simulink model "single_phase_five_level_CHB"  (R2022b)
settings: Solver=ode45  StartTime=0.0  StopTime=0.02  MaxStep=1e-5  RelTol=1e-4  EnableMultiTasking=on
libraries: spsIGBTDiodeLib x8, simulink x4, spsDCVoltageSourceLib x2, spsCurrentMeasurementLib x1, spsSeriesRLCBranchLib x1, spsTHDLib x1, spsVoltageMeasurementLib x1, sps_lib x1
settings Model: Creator=OLIVIA  LastModifiedBy=ugochukwu
settings SolverCC: AlgebraicLoopSolver=TrustRegion
settings DataIOCC: LimitDataPoints=on  SaveFormat=Array  ReturnWorkspaceOutputs=off
settings OptimizationCC: LifeSpan=inf
settings DebuggingCC: SolverPrmCheckMsg=warning  UnconnectedInputMsg=warning  UnconnectedOutputMsg=warning  UnconnectedLineMsg=warning  SFUnexpectedBacktrackingDiag=warning  SFNoUnconditionalDefaultTransitionDiag=warning  SFExecutionAtInitializationDiag=none  SFMachineParentedDataDiag=warning  ArithmeticOperatorsInVariantConditions=warning
settings HardwareCC: ProdBitPerPointer=32  ProdBitPerSizeT=32  ProdBitPerPtrDiffT=32  ProdLargestAtomicFloat=None  ProdIntDivRoundTo=Undefined  ProdEndianess=Unspecified  ProdWordSize=32  ProdHWDeviceType=32-bit Generic
settings ModelReferenceCC: PropagateSignalLabelsOutOfModel=off
settings SFSimCC: SimUseLocalCustomCode=off  CustomCodeUndefinedFunction=UseInterfaceOnly
settings RTWCC: RTWUseLocalCustomCode=off
settings CodeAppCC: StateflowObjectComments=on
settings GRTTargetCC: TargetLangStandard=C89/C90 (ANSI)
settings ConfigComp: CovMetricSettings=dw  CovSaveCumulativeToWorkspaceVar=on  CovSaveSingleToWorkspaceVar=on  CovExternalEMLEnable=off  CovSFcnEnable=off
settings SimscapeCC: SimscapeNormalizeSystem=off

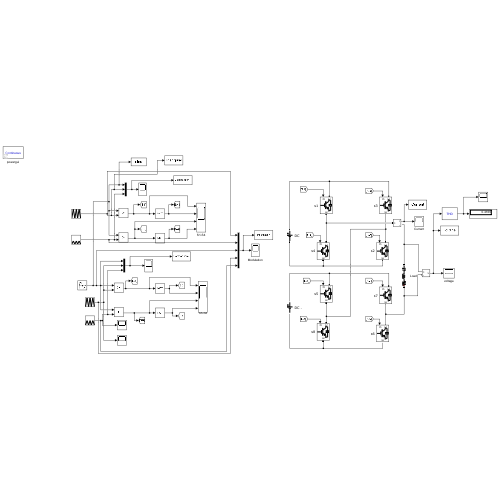
[thumbnail: Simulink's stored preview of the top-level diagram]
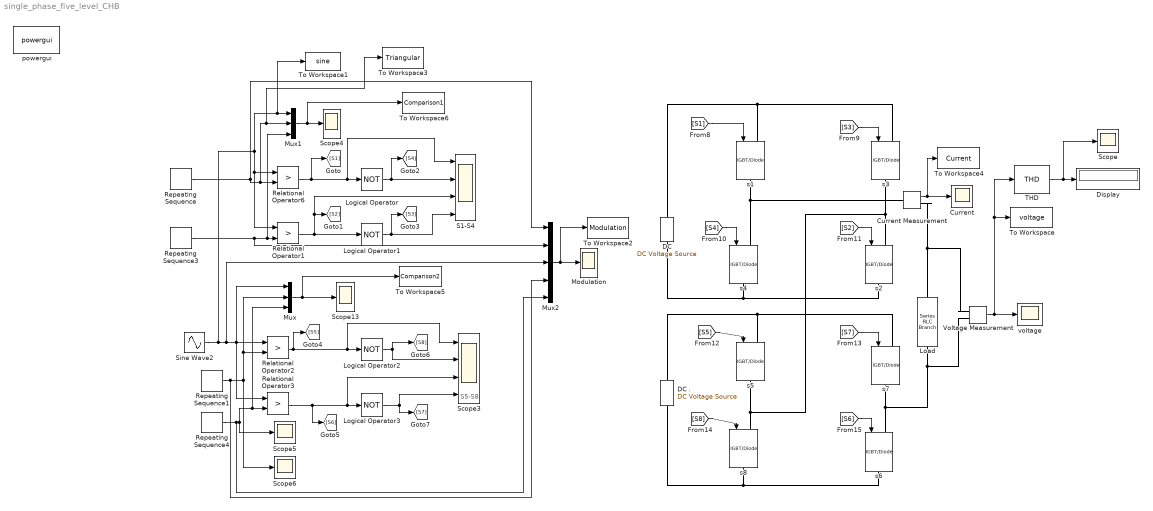
== system single_phase_five_level_CHB ==
  note: S5-S8
  Current : Scope
  Current Measurement : spsCurrentMeasurementLib/Current Measurement  PhasorSimulation=off  OutputType=Complex  PSBequivalent=0
  DC : spsDCVoltageSourceLib/DC Voltage Source  Amplitude=110  Measurements=None
  DC . : spsDCVoltageSourceLib/DC Voltage Source  Amplitude=110  Measurements=None
  Display : Display
  Load : spsSeriesRLCBranchLib/Series RLC Branch  LConnTagsString=__new0  RConnTagsString=__new0  BranchType=RLC  Resistance=100  Inductance=2e-3  SetiL0=off  InitialCurrent=0  Capacitance=1e-6  Setx0=off  InitialVoltage=0  Measurements=Branch voltage
  Logical Operator{,1..3} (4 alike) : Logic  Operator=NOT  AllPortsSameDT=off  OutDataTypeStr=boolean
  Modulation : Scope
  Mux : Mux  Inputs=3
  Mux1 : Mux  Inputs=3
  Mux2 : Mux  Inputs=5
  Relational Operator{1..3,6} (4 alike) : RelationalOperator  Operator=>  OutDataTypeStr=boolean  InputSameDT=off
  Repeating Sequence : simulink/Sources/Repeating Sequence  rep_seq_t=[0 1/4000 1/2000]  rep_seq_y=[1 1.5 1 ]
  Repeating Sequence1 : simulink/Sources/Repeating Sequence  rep_seq_t=[0 1/4000 1/2000]  rep_seq_y=[0.5 1 0.5]
  Repeating Sequence3 : simulink/Sources/Repeating Sequence  rep_seq_t=[0 1/4000 1/2000]  rep_seq_y=[-1.5 -1 -1.5 ]
  Repeating Sequence4 : simulink/Sources/Repeating Sequence  rep_seq_t=[0 1/4000 1/2000]  rep_seq_y=[-1 -0.5 -1]
  S1-S4 : Scope  NumInputPorts=4
  Scope{,4..6,13} (5 alike) : Scope
  Scope3 : Scope  NumInputPorts=4
  Sine Wave2 : Sin  Amplitude=1.4  Frequency=2*50*pi  SampleTime=0
  THD : spsTHDLib/THD  Freq=50  Ts=0
  To Workspace : ToWorkspace  VariableName=voltage  SaveFormat=Timeseries  SampleTime=-1
  To Workspace1 : ToWorkspace  VariableName=sine  SaveFormat=Timeseries  SampleTime=-1
  To Workspace2 : ToWorkspace  VariableName=Modulation  SaveFormat=Timeseries  SampleTime=-1
  To Workspace3 : ToWorkspace  VariableName=Triangular  SaveFormat=Timeseries  SampleTime=-1
  To Workspace4 : ToWorkspace  VariableName=Current  SaveFormat=Timeseries  SampleTime=-1
  To Workspace5 : ToWorkspace  VariableName=Comparison2  SaveFormat=Timeseries  SampleTime=-1
  To Workspace6 : ToWorkspace  VariableName=Comparison1  SaveFormat=Timeseries  SampleTime=-1
  Voltage Measurement : spsVoltageMeasurementLib/Voltage Measurement  PhasorSimulation=off  OutputType=Complex  PSBequivalent=0
  powergui : sps_lib/powergui  Priority=1  SimulationMode=Continuous  SampleTime=50e-6  frequency=60  Iterations=50  frequencyindice=0  Pbase=100e6  ErrMax=1e-4  UnitsV=kV  UnitsW=MW  buscounter=0  FunctionMessages=off  echomessages=off  EnableUseOfTLC=off  CurrentSourceSwitches=on  DisableSnubberDevices=off  DisableRonSwitches=off  DisableVfSwitches=off  DisplayEquations=off  AutomaticDiscreteSolvers=off  SolverType=Tustin  Interpol=off  ExternalGateDelay=off  methode=off  Ts=0  x0status=blocks  SPID=off  SwTol=0  HookPort=off  NonlinearTolerance=1e-4  nMaxIteration=100  ContinueOnMaxIteration=off  RestoreLinks=warning  ResistiveCurrentMeasurement=off  Frange=[0:2:500]  Ylog=off  Xlog=on  ShowGrid=off  save=off  variable=ZData  structure=0  ZoomFFT=off  StartTime=0.0  cycles=1  DisplayStyle=1  fundamental=60  FreqAxis=off  MaxFrequency=1000  frequencyindicesteady=1  RmsSteady=1  display=off
  s{1..8} (8 alike) : spsIGBTDiodeLib/IGBT//Diode  Ron=1e-3  Rs=1e5  Cs=inf  Measurements=off
  voltage : Scope
  wires:
  Relational Operator6/1 -> Logical Operator/1, S1-S4/1, [S1]
  Relational Operator1/1 -> S1-S4/3, [S2], Logical Operator1/1
  Logical Operator1/1 -> [S3], S1-S4/4
  Logical Operator/1 -> S1-S4/2, [S4]
  Relational Operator2/1 -> Logical Operator2/1, Scope3/1, [S5]
  Relational Operator3/1 -> [S6], Logical Operator3/1, Scope3/3
  Logical Operator3/1 -> [S7], Scope3/4
  Logical Operator2/1 -> Scope3/2, [S8]
  Sine Wave2/1 -> Mux1/1, To Workspace1/1, Relational Operator6/1, Relational Operator1/1, Mux2/3, Mux/1, Relational Operator3/1, Relational Operator2/1
  Repeating Sequence1/1 -> Mux2/4, Scope6/1, Relational Operator2/2, Mux/2
  Repeating Sequence3/1 -> Mux2/2, Mux1/3, Relational Operator1/2
  Repeating Sequence4/1 -> Mux2/5, Scope5/1, Mux/3, Relational Operator3/2
  Mux/1 -> To Workspace5/1, Scope13/1
  Mux1/1 -> To Workspace6/1, Scope4/1
  [S1] -> s1/1
  [S3] -> s3/1
  [S4] -> s4/1
  [S2] -> s2/1
  [S5] -> s5/1
  [S7] -> s7/1
  [S8] -> s8/1
  [S6] -> s6/1
  Voltage Measurement/1 -> THD/1, To Workspace/1, voltage/1
  Mux2/1 -> To Workspace2/1, Modulation/1
  Repeating Sequence/1 -> Mux1/2, To Workspace3/1, Relational Operator6/2, Mux2/1
  THD/1 -> Display/1, Scope/1
  Current Measurement/1 -> Current/1, To Workspace4/1
  connections:
  s1/RConn1 -- s4/LConn1 -- Current Measurement/LConn1
  s2/LConn1 -- s5/RConn1 -- s8/LConn1 -- s3/RConn1
  DC/RConn1 -- s3/LConn1 -- s1/LConn1
  DC/LConn1 -- s2/RConn1 -- s4/RConn1
  DC ./RConn1 -- s7/LConn1 -- s5/LConn1
  DC ./LConn1 -- s6/RConn1 -- s8/RConn1
  Load/LConn1 -- s6/LConn1 -- s7/RConn1 -- Voltage Measurement/LConn2
  Current Measurement/RConn1 -- Voltage Measurement/LConn1 -- Load/RConn1
